simulink model "track_vehicle_EKF1"  (R2017b)
settings: Solver=ode45  StartTime=0.0  StopTime=300  FixedStep=0.1  RelTol=1e-3  EnableMultiTasking=on
PreLoadFcn:
  | RTWConfigurationCB('preloadfcn', bdroot);
InitFcn:
  | parameterVehicle
  | parameterGNC
StopFcn:
  | myAnimation(xActEst,yActEst,thetaActEst,X_array,Y_array,rp1,rp2)
  | myStopFcn2sim(xActEst,yActEst,X_array,Y_array,rp1,rp2)
undefined symbols (not defined in the file): bDR, dcArrayC, DiscIntNeverNeededParam, Earth, eTickDR, KP1, KP2, rNominalDR, rp1, rp2, Tau1, Tau2, TauEncoderDR, Tsample, TsampleEncoderDR, Vcom, wArrayC, WGS84, X, X_array, Y, Y_array
libraries: simulink x12, robotlib x8, aerolibtransform2 x1, dspsigops x1, aerolibanimutils x1
CloseFcn:
  | rtwprivate ssgencode ModelCloseRequest track_vehicle6_v2
settings Model: Creator=Dogan  LastModifiedBy=ayushi
settings DataIOCC: LimitDataPoints=on  SaveFormat=Array  SignalLoggingSaveFormat=ModelDataLogs
settings OptimizationCC: ExpressionDepthLimit=2147483647  InitFltsAndDblsToZero=on  LifeSpan=inf
settings DebuggingCC: SaveWithParameterizedLinksMsg=none  UnderspecifiedInitializationDetection=Classic  MergeDetectMultiDrivingBlocksExec=none  SignalResolutionControl=TryResolveAllWithWarning  SolverPrmCheckMsg=warning  MultiTaskDSMMsg=warning  MultiTaskCondExecSysMsg=none  ParameterPrecisionLossMsg=none  FcnCallInpInsideContextMsg=warning  StateNameClashWarn=warning  SFUnexpectedBacktrackingDiag=warning  SFNoUnconditionalDefaultTransitionDiag=warning  SFExecutionAtInitializationDiag=none
settings HardwareCC: ProdBitPerLong=64  ProdLargestAtomicFloat=None  ProdHWDeviceType=Intel->x86-64  TargetHWDeviceType=32-bit Generic
settings ModelReferenceCC: PropagateSignalLabelsOutOfModel=off
settings SFSimCC: SimParseCustomCode=off
settings RTWCC: Description=Generic Real-Time Target
settings CodeAppCC: GenerateComments=off  SimulinkBlockComments=off
settings GRTTargetCC: TargetLangStandard=C89/C90 (ANSI)  GeneratePreprocessorConditionals=Disable all
settings ConfigComp: CovMetricSettings=dw  CovHtmlReporting=on  CovSaveCumulativeToWorkspaceVar=on  CovSaveSingleToWorkspaceVar=on  CovExternalEMLEnable=off

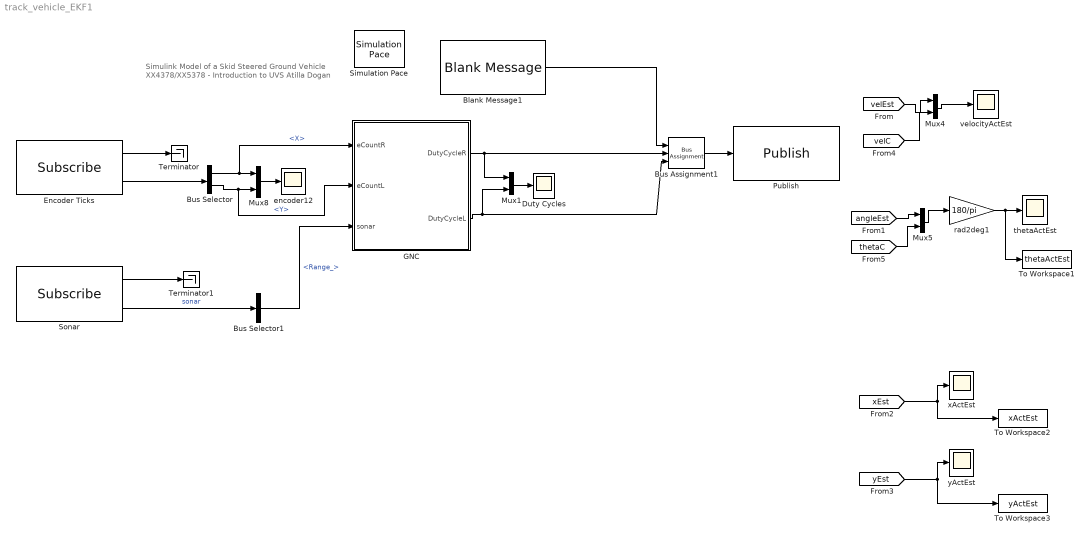
== system track_vehicle_EKF1 ==
  note: Simulink Model of a Skid Steered Ground Vehicle
      | XX4378/XX5378 - Introduction to UVS
      | Atilla Dogan
  Blank Message1 : robotlib/Blank Message  SourceLibraryInfo=This block requires Robotics System Toolbox  messageType=geometry_msgs/Point  SampleTime=inf
      settings: SourceProductBaseCode=RO
  Bus Assignment1 : BusAssignment  AssignedSignals=X,Y
  Bus Selector : BusSelector  OutputSignals=Point.X,Point.Y
  Bus Selector1 : BusSelector  OutputSignals=Range_
  Duty Cycles : Scope
  Encoder Ticks : robotlib/Subscribe  SourceLibraryInfo=This block requires Robotics System Toolbox  topicSource=Select from ROS network  topic=/enc  messageType=geometry_msgs/PointStamped  sampleTime=-1  messageQueueLength=1
      settings: SourceProductBaseCode=RO
  GNC : Subsystem
  Mux{1,4..5,8} (4 alike) : Mux  Inputs=2
  Publish : robotlib/Publish  SourceLibraryInfo=This block requires Robotics System Toolbox  topicSource=Select from ROS network  topic=/cmd_pwm  messageType=geometry_msgs/Point  messageQueueLength=10
      settings: SourceProductBaseCode=RO
  Simulation Pace : aerolibanimutils/Simulation Pace  SimulationPace=1  SleepMode=MATLAB Thread  OutputPaceError=off  SampleTime=1/30
  Sonar : robotlib/Subscribe  SourceLibraryInfo=This block requires Robotics System Toolbox  topicSource=Select from ROS network  topic=/mavros/distance_sensor/hrlv_ez4_pub  messageType=sensor_msgs/Range  sampleTime=-1  messageQueueLength=1
      settings: SourceProductBaseCode=RO
  Terminator : Terminator
  Terminator1 : Terminator
  To Workspace1 : ToWorkspace  VariableName=thetaActEst  SaveFormat=Structure With Time  SampleTime=-1
  To Workspace2 : ToWorkspace  VariableName=xActEst  SaveFormat=Structure With Time  SampleTime=-1
  To Workspace3 : ToWorkspace  VariableName=yActEst  SaveFormat=Structure With Time  SampleTime=-1
  encoder12 : Scope
  rad2deg1 : Gain  Gain=180/pi
  thetaActEst : Scope
  velocityActEst : Scope
  xActEst : Scope
  yActEst : Scope
  wires:
  GNC/1(DutyCycleR) -> Bus Assignment1/2, Mux1/1
  GNC/2(DutyCycleL) -> Bus Assignment1/3, Mux1/2
  Mux1/1 -> Duty Cycles/1
  Mux4/1 -> velocityActEst/1
  [velEst] -> Mux4/1
  rad2deg1/1 -> To Workspace1/1, thetaActEst/1
  Mux5/1 -> rad2deg1/1
  [angleEst] -> Mux5/1
  [xEst] -> xActEst/1, To Workspace2/1
  [yEst] -> yActEst/1, To Workspace3/1
  [velC] -> Mux4/2
  [thetaC] -> Mux5/2
  Encoder Ticks/2 -> Bus Selector/1
  Bus Selector/2 -> GNC/2(eCountL), Mux8/2  "<Y>"
  Bus Selector/1 -> GNC/1(eCountR), Mux8/1  "<X>"
  Mux8/1 -> encoder12/1
  Encoder Ticks/1 -> Terminator/1
  Blank Message1/1 -> Bus Assignment1/1
  Bus Assignment1/1 -> Publish/1
  Sonar/1 -> Terminator1/1
  Sonar/2 -> Bus Selector1/1  "sonar"
  Bus Selector1/1 -> GNC/3(sonar)  "<Range_>"

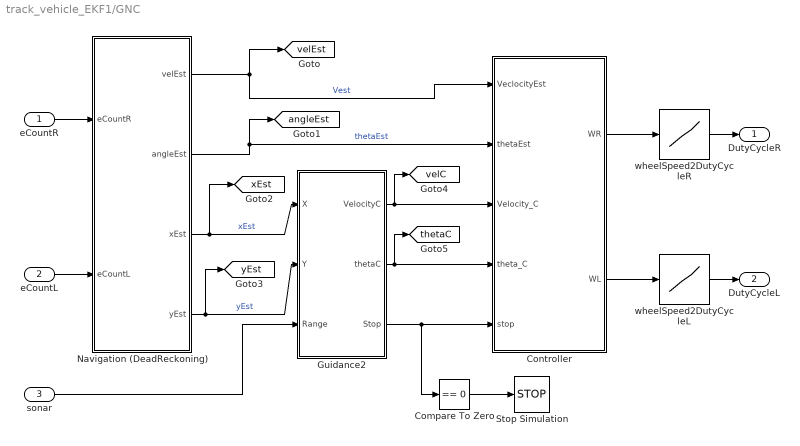
== system track_vehicle_EKF1/GNC ==
  eCountR : Inport
  eCountL : Inport  Port=2
  sonar : Inport  Port=3
  Compare To Zero : simulink/Logic and Bit Operations/Compare To Zero  relop===  OutDataTypeStr=boolean
  Controller : Subsystem
  Guidance2 : Subsystem
  Navigation (DeadReckoning) : Subsystem
  Stop Simulation : Stop
  wheelSpeed2DutyCycleL : Lookup  InputValues=wArrayC  Table=dcArrayC  LookUpMeth=Use Input Nearest
  wheelSpeed2DutyCycleR : Lookup  InputValues=wArrayC  Table=dcArrayC  LookUpMeth=Use Input Nearest
  DutyCycleR : Outport
  DutyCycleL : Outport  Port=2
  tag scope: angleEst=global, thetaC=global, velC=global, velEst=global, xEst=global, yEst=global
  wires:
  Guidance2/3(Stop) -> Compare To Zero/1, Controller/5(stop)
  Controller/1(WR) -> wheelSpeed2DutyCycleR/1
  Navigation (DeadReckoning)/4(yEst) -> [yEst], Guidance2/2(Y)  "yEst"
  Navigation (DeadReckoning)/3(xEst) -> Guidance2/1(X), [xEst]  "xEst"
  Navigation (DeadReckoning)/2(angleEst) -> Controller/2(thetaEst), [angleEst]  "thetaEst"
  Navigation (DeadReckoning)/1(velEst) -> Controller/1(VeclocityEst), [velEst]  "Vest"
  eCountL/1 -> Navigation (DeadReckoning)/2(eCountL)
  eCountR/1 -> Navigation (DeadReckoning)/1(eCountR)
  Guidance2/1(VelocityC) -> Controller/3(Velocity_C), [velC]
  Guidance2/2(thetaC) -> Controller/4(theta_C), [thetaC]
  wheelSpeed2DutyCycleR/1 -> DutyCycleR/1
  Controller/2(WL) -> wheelSpeed2DutyCycleL/1
  wheelSpeed2DutyCycleL/1 -> DutyCycleL/1
  Compare To Zero/1 -> Stop Simulation/1
  sonar/1 -> Guidance2/3(Range)

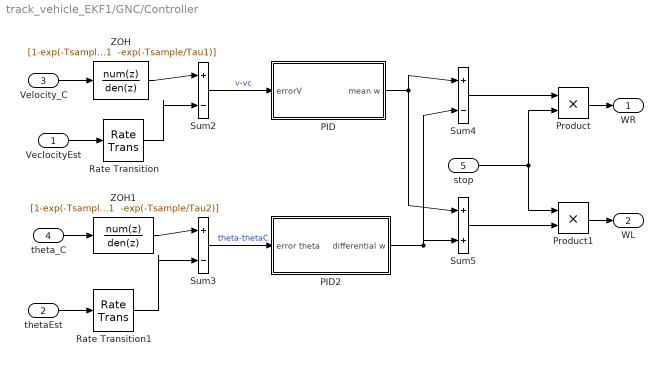
== system track_vehicle_EKF1/GNC/Controller ==
  VeclocityEst : Inport
  thetaEst : Inport  Port=2
  Velocity_C : Inport  Port=3
  theta_C : Inport  Port=4
  stop : Inport  Port=5
  PID : Subsystem
  PID2 : Subsystem
  Product : Product  RndMeth=Zero
  Product1 : Product  RndMeth=Zero
  Rate Transition : RateTransition  Deterministic=off
  Rate Transition1 : RateTransition  Deterministic=off
  Sum2 : Sum  Inputs=|+|-|  SampleTime=Tsample
  Sum3 : Sum  Inputs=|+|-|  SampleTime=Tsample
  Sum4 : Sum  Inputs=+|-
  Sum5 : Sum  Inputs=+|+
  ZOH : DiscreteTransferFcn  Numerator=[1-exp(-Tsample/Tau1)]  Denominator="[1  -exp(-Tsample/Tau1)]"  SampleTime=Tsample
  ZOH1 : DiscreteTransferFcn  Numerator=[1-exp(-Tsample/Tau2)]  Denominator="[1  -exp(-Tsample/Tau2)]"  SampleTime=Tsample
  WR : Outport
  WL : Outport  Port=2
  wires:
  Product1/1 -> WL/1
  Product/1 -> WR/1
  Sum5/1 -> Product1/2
  stop/1 -> Product/2, Product1/1
  Sum4/1 -> Product/1
  PID2/1(differential w) -> Sum5/2, Sum4/2
  PID/1(mean w) -> Sum5/1, Sum4/1
  theta_C/1 -> ZOH1/1
  thetaEst/1 -> Rate Transition1/1
  Velocity_C/1 -> ZOH/1
  VeclocityEst/1 -> Rate Transition/1
  Sum2/1 -> PID/1(errorV)  "v-vc"
  Sum3/1 -> PID2/1(error theta)  "theta-thetaC"
  ZOH/1 -> Sum2/1
  Rate Transition/1 -> Sum2/2
  ZOH1/1 -> Sum3/1
  Rate Transition1/1 -> Sum3/2

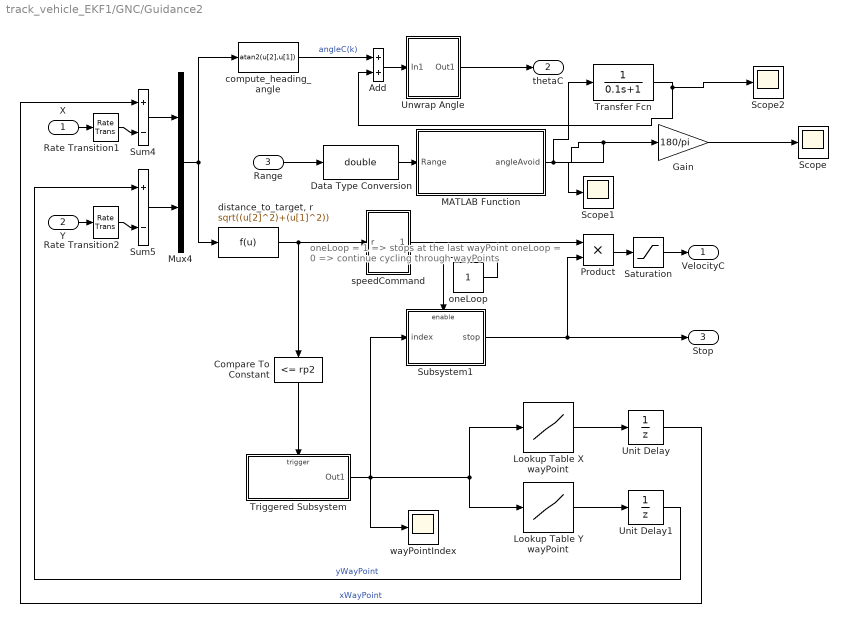
== system track_vehicle_EKF1/GNC/Guidance2 ==
  note: oneLoop = 1 => stops at the last wayPoint
      | oneLoop = 0 => continue cycling through wayPoints
  X : Inport
  Y : Inport  Port=2
  Range : Inport  Port=3
  Add : Sum
  Compare To Constant : simulink/Logic and Bit Operations/Compare To Constant  relop=<=  const=rp2  OutDataTypeStr=uint8  ZeroCross=off
  Data Type Conversion : DataTypeConversion  OutDataTypeStr=double
  Gain : Gain  Gain=180/pi
  Lookup Table X wayPoint : Lookup  InputValues=[1:length(X_array)]  Table=X_array  LookUpMeth=Interpolation-Use End Values  OutDataTypeStr=double
  Lookup Table Y wayPoint : Lookup  InputValues=[1:length(Y_array)]  Table=Y_array  LookUpMeth=Interpolation-Use End Values  OutDataTypeStr=double
  MATLAB Function : MATLAB Function  TreatAsAtomicUnit=on
  Mux4 : Mux  Inputs=2
  Product : Product  RndMeth=Zero
  Rate Transition1 : RateTransition
  Rate Transition2 : RateTransition
  Saturation : Saturate  UpperLimit=Vcom  LowerLimit=0  SampleTime=Tsample
  Scope : Scope
  Scope1 : Scope
  Scope2 : Scope
  Subsystem1 : Subsystem
  Sum4 : Sum  Inputs=|+|-|
  Sum5 : Sum  Inputs=|+|-|
  Transfer Fcn : TransferFcn  Denominator=[0.1 1]
  Triggered Subsystem : Subsystem  TreatAsAtomicUnit=on
  Unit Delay : UnitDelay  SampleTime=Tsample
  Unit Delay1 : UnitDelay  SampleTime=Tsample
  Unwrap Angle : Subsystem
  compute_heading_angle : Fcn  Expr=atan2(u[2],u[1])  SampleTime=Tsample
  "distance_to_target, r" : Fcn  Expr=sqrt((u[2]^2)+(u[1]^2))  SampleTime=Tsample
  oneLoop : Constant  OutDataTypeStr=uint32  SampleTime=Tsample
  speedCommand : Subsystem
  wayPointIndex : Scope
  VelocityC : Outport
  thetaC : Outport  Port=2
  Stop : Outport  Port=3
  wires:
  speedCommand/1(Vdes) -> Product/1
  compute_heading_angle/1 -> Add/1  "angleC(k)"
  Sum4/1 -> Mux4/1
  "distance_to_target, r"/1 -> speedCommand/1(r), Compare To Constant/1
  Mux4/1 -> "distance_to_target, r"/1, compute_heading_angle/1
  Lookup Table X wayPoint/1 -> Unit Delay/1
  Lookup Table Y wayPoint/1 -> Unit Delay1/1
  X/1 -> Rate Transition1/1
  Y/1 -> Rate Transition2/1
  Sum5/1 -> Mux4/2
  Compare To Constant/1 -> Triggered Subsystem/Trigger
  Triggered Subsystem/1(Out1) -> Subsystem1/1(index), wayPointIndex/1, Lookup Table X wayPoint/1, Lookup Table Y wayPoint/1
  Unit Delay/1 -> Sum4/1  "xWayPoint"
  Unit Delay1/1 -> Sum5/1  "yWayPoint"
  Saturation/1 -> VelocityC/1
  Unwrap Angle/1(Out1) -> thetaC/1
  Rate Transition1/1 -> Sum4/2
  Rate Transition2/1 -> Sum5/2
  Product/1 -> Saturation/1
  Subsystem1/1(stop) -> Product/2, Stop/1
  oneLoop/1 -> Subsystem1/Enable
  Gain/1 -> Scope/1
  Data Type Conversion/1 -> MATLAB Function/1(Range)
  Range/1 -> Data Type Conversion/1
  Add/1 -> Unwrap Angle/1(In1)
  MATLAB Function/1(angleAvoid) -> Transfer Fcn/1, Scope1/1, Gain/1
  Transfer Fcn/1 -> Scope2/1, Add/2

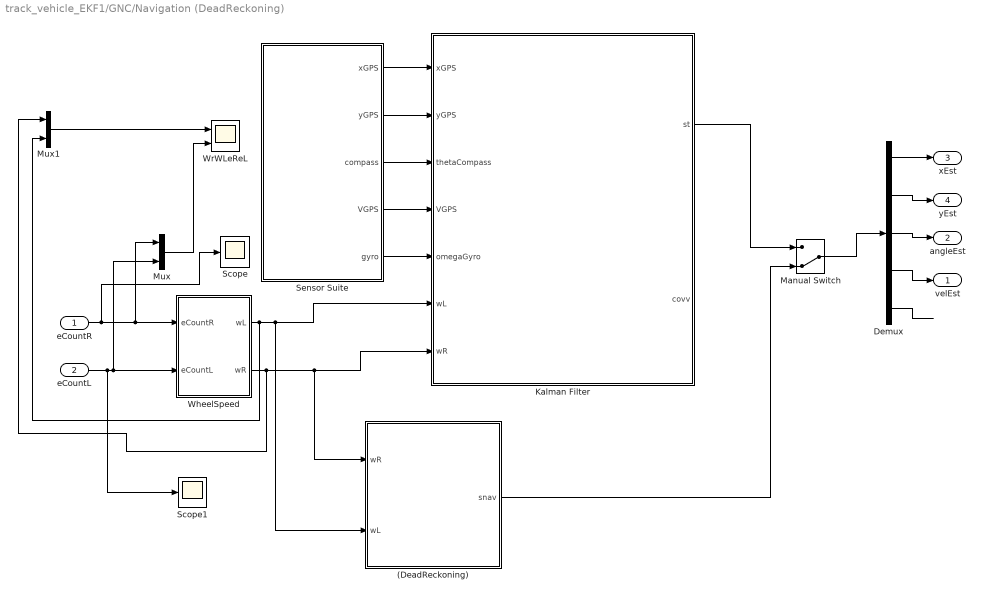
== system track_vehicle_EKF1/GNC/Navigation (DeadReckoning) ==
  eCountR : Inport
  eCountL : Inport  Port=2
  (DeadReckoning) : Subsystem
  Demux : Demux  Outputs=5
  Kalman Filter : MATLAB Function  TreatAsAtomicUnit=on  SystemSampleTime=Tsample
  Manual Switch : ManualSwitch  CurrentSetting=0
  Mux : Mux  Inputs=2
  Mux1 : Mux  Inputs=2
  Scope : Scope
  Scope1 : Scope
  Sensor Suite : Subsystem
  WheelSpeed : Subsystem
  WrWLeReL : Scope  NumInputPorts=2
  velEst : Outport
  angleEst : Outport  Port=2
  xEst : Outport  Port=3
  yEst : Outport  Port=4
  wires:
  WheelSpeed/2(wR) -> Mux1/1, (DeadReckoning)/1(wR), Kalman Filter/7(wR)
  eCountL/1 -> Scope1/1, WheelSpeed/2(eCountL), Mux/2
  eCountR/1 -> Scope/1, Mux/1, WheelSpeed/1(eCountR)
  Sensor Suite/5(gyro) -> Kalman Filter/5(omegaGyro)
  Demux/5 -> ?
  Demux/1 -> xEst/1
  Demux/2 -> yEst/1
  Demux/3 -> angleEst/1
  Demux/4 -> velEst/1
  Kalman Filter/1(st) -> Manual Switch/1
  (DeadReckoning)/1(snav) -> Manual Switch/2
  Manual Switch/1 -> Demux/1
  WheelSpeed/1(wL) -> Kalman Filter/6(wL), (DeadReckoning)/2(wL), Mux1/2
  Mux/1 -> WrWLeReL/2
  Mux1/1 -> WrWLeReL/1
  Sensor Suite/1(xGPS) -> Kalman Filter/1(xGPS)
  Sensor Suite/2(yGPS) -> Kalman Filter/2(yGPS)
  Sensor Suite/3(compass) -> Kalman Filter/3(thetaCompass)
  Sensor Suite/4(VGPS) -> Kalman Filter/4(VGPS)

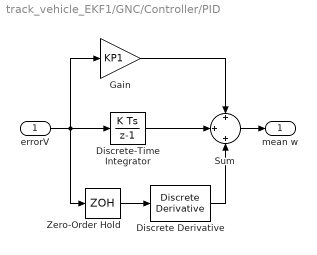
== system track_vehicle_EKF1/GNC/Controller/PID ==
  errorV : Inport
  Discrete Derivative : simulink/Discrete/Discrete Derivative  gainval=KD1  ICPrevScaledInput=0.0  InputProcessing=Inherited  OutMin=[]  OutMax=[]  OutDataType=sfix(16)  OutScaling=2^-10  DoSatur=off
  Discrete-Time Integrator : DiscreteIntegrator  gainval=KI1  SampleTime=Tsample  ICPrevOutput=DiscIntNeverNeededParam  ICPrevScaledInput=DiscIntNeverNeededParam
  Gain : Gain  Gain=KP1  SampleTime=Tsample
  Sum : Sum  Inputs=+|+|+
  Zero-Order Hold : ZeroOrderHold  SampleTime=Tsample
  mean w : Outport
  wires:
  Discrete Derivative/1 -> Sum/3
  Zero-Order Hold/1 -> Discrete Derivative/1
  Discrete-Time Integrator/1 -> Sum/2
  Gain/1 -> Sum/1
  errorV/1 -> Discrete-Time Integrator/1, Gain/1, Zero-Order Hold/1
  Sum/1 -> mean w/1

== system track_vehicle_EKF1/GNC/Controller/PID2 ==
  error theta : Inport
  Discrete Derivative1 : simulink/Discrete/Discrete Derivative  gainval=KD2  ICPrevScaledInput=0.0  InputProcessing=Inherited  OutMin=[]  OutMax=[]  OutDataType=sfix(16)  OutScaling=2^-10  DoSatur=off
  Discrete-Time Integrator1 : DiscreteIntegrator  gainval=KI2  SampleTime=Tsample  ICPrevOutput=DiscIntNeverNeededParam  ICPrevScaledInput=DiscIntNeverNeededParam
  Gain1 : Gain  Gain=KP2  SampleTime=Tsample
  Sum1 : Sum  Inputs=+|+|+
  Zero-Order Hold1 : ZeroOrderHold  SampleTime=Tsample
  differential w : Outport
  wires:
  Discrete Derivative1/1 -> Sum1/3
  Zero-Order Hold1/1 -> Discrete Derivative1/1
  error theta/1 -> Gain1/1, Discrete-Time Integrator1/1, Zero-Order Hold1/1
  Discrete-Time Integrator1/1 -> Sum1/2
  Gain1/1 -> Sum1/1
  Sum1/1 -> differential w/1

== system track_vehicle_EKF1/GNC/Guidance2/Subsystem1 ==
  note: NAND = TRUE
      | if at least one input is FALSE
  index : Inport
  Enable : EnablePort
  Compare To Constant1 : simulink/Logic and Bit Operations/Compare To Constant  relop===  const=1  OutDataTypeStr=uint8  ZeroCross=off
  Compare To Constant2 : simulink/Logic and Bit Operations/Compare To Constant  relop===  const=length(X_array)  OutDataTypeStr=uint8  ZeroCross=off
  Logical Operator1 : Logic  Operator=NAND  IconShape=distinctive  AllPortsSameDT=off  OutDataTypeStr=boolean
  Triggered Subsystem2 : Subsystem  TreatAsAtomicUnit=on
  stop : Outport  OutputWhenDisabled=reset  InitialOutput=[1]
  wires:
  Logical Operator1/1 -> stop/1
  index/1 -> Compare To Constant1/1, Compare To Constant2/1
  Compare To Constant1/1 -> Logical Operator1/1
  Triggered Subsystem2/1(Out1) -> Logical Operator1/2
  Compare To Constant2/1 -> Triggered Subsystem2/Trigger

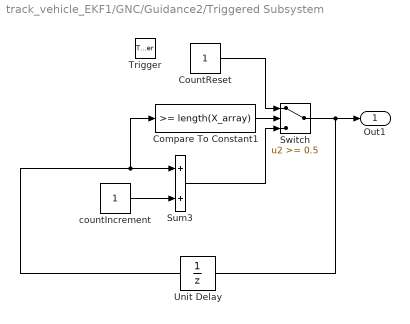
== system track_vehicle_EKF1/GNC/Guidance2/Triggered Subsystem ==
  Trigger : TriggerPort  VariantControl=(inherit)
  Compare To Constant1 : simulink/Logic and Bit Operations/Compare To Constant  relop=>=  const=length(X_array)  OutDataTypeStr=uint8  ZeroCross=off
  CountReset : Constant  OutDataTypeStr=uint32  SampleTime=-1
  Sum3 : Sum  OutDataTypeStr=uint32
  Switch : Switch  Threshold=0.5
  Unit Delay : UnitDelay  InitialCondition=1  SampleTime=-1
  countIncrement : Constant  OutDataTypeStr=uint32  SampleTime=-1
  Out1 : Outport  OutDataTypeStr=uint32  InitialOutput=1
  wires:
  countIncrement/1 -> Sum3/2
  Unit Delay/1 -> Sum3/1, Compare To Constant1/1
  Compare To Constant1/1 -> Switch/2
  Switch/1 -> Out1/1, Unit Delay/1
  CountReset/1 -> Switch/1
  Sum3/1 -> Switch/3

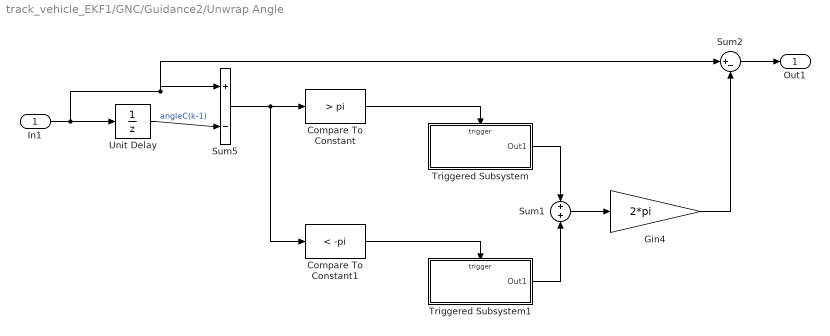
== system track_vehicle_EKF1/GNC/Guidance2/Unwrap Angle ==
  In1 : Inport
  Compare To Constant : simulink/Logic and Bit Operations/Compare To Constant  relop=>  const=pi  OutDataTypeStr=uint8  ZeroCross=off
  Compare To Constant1 : simulink/Logic and Bit Operations/Compare To Constant  relop=<  const=-pi  OutDataTypeStr=uint8  ZeroCross=off
  Gin4 : Gain  Gain=2*pi  OutDataTypeStr=double  SampleTime=Tsample
  Sum1 : Sum  Inputs=+|+
  Sum2 : Sum  Inputs=|+-
  Sum5 : Sum  Inputs=|+|-|
  Triggered Subsystem : Subsystem  TreatAsAtomicUnit=on
  Triggered Subsystem1 : Subsystem  TreatAsAtomicUnit=on
  Unit Delay : UnitDelay  SampleTime=Tsample
  Out1 : Outport
  wires:
  In1/1 -> Unit Delay/1, Sum5/1, Sum2/1
  Unit Delay/1 -> Sum5/2  "angleC(k-1)"
  Sum5/1 -> Compare To Constant/1, Compare To Constant1/1
  Compare To Constant1/1 -> Triggered Subsystem1/Trigger
  Compare To Constant/1 -> Triggered Subsystem/Trigger
  Triggered Subsystem/1(Out1) -> Sum1/1
  Triggered Subsystem1/1(Out1) -> Sum1/2
  Sum1/1 -> Gin4/1
  Sum2/1 -> Out1/1
  Gin4/1 -> Sum2/2

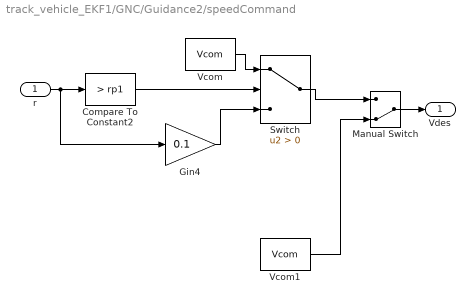
== system track_vehicle_EKF1/GNC/Guidance2/speedCommand ==
  r : Inport
  Compare To Constant2 : simulink/Logic and Bit Operations/Compare To Constant  relop=>  const=rp1  OutDataTypeStr=uint8  ZeroCross=off
  Gin4 : Gain  Gain=0.1  SampleTime=Tsample
  Manual Switch : ManualSwitch  CurrentSetting=0
  Switch : Switch  Criteria=u2 > Threshold
  Vcom : Constant  Value=Vcom  SampleTime=Tsample
  Vcom1 : Constant  Value=Vcom  SampleTime=Tsample
  Vdes : Outport
  wires:
  Compare To Constant2/1 -> Switch/2
  Vcom/1 -> Switch/1
  Vcom1/1 -> Manual Switch/2
  Switch/1 -> Manual Switch/1
  Gin4/1 -> Switch/3
  r/1 -> Compare To Constant2/1, Gin4/1
  Manual Switch/1 -> Vdes/1

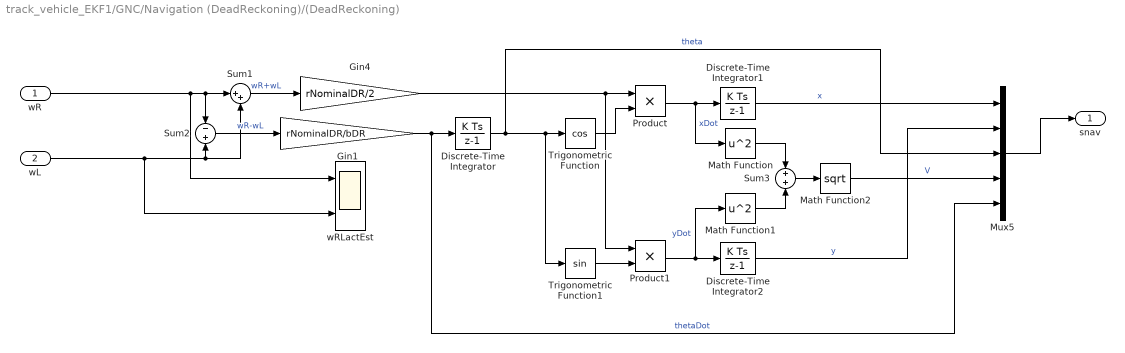
== system track_vehicle_EKF1/GNC/Navigation (DeadReckoning)/(DeadReckoning) ==
  wR : Inport
  wL : Inport  Port=2
  Discrete-Time Integrator : DiscreteIntegrator  SampleTime=TsampleEncoderDR  ICPrevOutput=DiscIntNeverNeededParam  ICPrevScaledInput=DiscIntNeverNeededParam
  Discrete-Time Integrator1 : DiscreteIntegrator  SampleTime=TsampleEncoderDR  ICPrevOutput=DiscIntNeverNeededParam  ICPrevScaledInput=DiscIntNeverNeededParam
  Discrete-Time Integrator2 : DiscreteIntegrator  SampleTime=TsampleEncoderDR  ICPrevOutput=DiscIntNeverNeededParam  ICPrevScaledInput=DiscIntNeverNeededParam
  Gin1 : Gain  Gain=rNominalDR/bDR  OutDataTypeStr=double
  Gin4 : Gain  Gain=rNominalDR/2  OutDataTypeStr=double
  Math Function : Math  Operator=square  SaturateOnIntegerOverflow=on
  Math Function1 : Math  Operator=square  SaturateOnIntegerOverflow=on
  Math Function2 : Math  Operator=sqrt  OutputSignalType=real  SaturateOnIntegerOverflow=on
  Mux5 : Mux  Inputs=5
  Product : Product  RndMeth=Zero
  Product1 : Product  RndMeth=Zero
  Sum1 : Sum  Inputs=|++
  Sum2 : Sum  Inputs=-|+
  Sum3 : Sum  Inputs=+|+
  Trigonometric Function : Trigonometry  Operator=cos  OutputSignalType=real
  Trigonometric Function1 : Trigonometry  OutputSignalType=real
  wRLactEst : Scope  NumInputPorts=2
  snav : Outport
  wires:
  wL/1 -> Sum2/2, Sum1/2, wRLactEst/2
  wR/1 -> Sum2/1, Sum1/1, wRLactEst/1
  Math Function2/1 -> Mux5/4  "V"
  Sum3/1 -> Math Function2/1
  Math Function1/1 -> Sum3/2
  Math Function/1 -> Sum3/1
  Discrete-Time Integrator2/1 -> Mux5/2  "y"
  Discrete-Time Integrator1/1 -> Mux5/1  "x"
  Product1/1 -> Math Function1/1, Discrete-Time Integrator2/1  "yDot"
  Product/1 -> Math Function/1, Discrete-Time Integrator1/1  "xDot"
  Trigonometric Function1/1 -> Product1/2
  Gin4/1 -> Product1/1, Product/1
  Trigonometric Function/1 -> Product/2
  Discrete-Time Integrator/1 -> Mux5/3, Trigonometric Function1/1, Trigonometric Function/1  "theta"
  Gin1/1 -> Mux5/5, Discrete-Time Integrator/1  "thetaDot"
  Sum2/1 -> Gin1/1  "wR-wL"
  Sum1/1 -> Gin4/1  "wR+wL"
  Mux5/1 -> snav/1

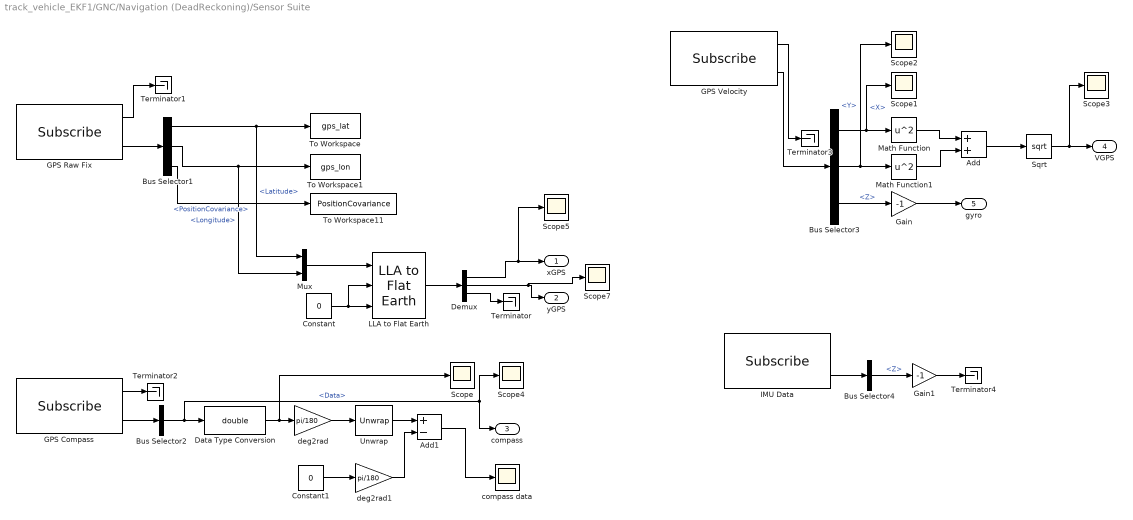
== system track_vehicle_EKF1/GNC/Navigation (DeadReckoning)/Sensor Suite ==
  " GPS Compass" : robotlib/Subscribe  SourceLibraryInfo=This block requires Robotics System Toolbox  topicSource=Select from ROS network  topic=/mavros/global_position/compass_hdg  messageType=std_msgs/Float64  sampleTime=-1  messageQueueLength=1
      settings: SourceProductBaseCode=RO
  Add : Sum  Inputs=2
  Add1 : Sum  Inputs=+-
  Bus Selector1 : BusSelector  OutputSignals=Latitude,Longitude,PositionCovariance
  Bus Selector2 : BusSelector  OutputSignals=Data
  Bus Selector3 : BusSelector  OutputSignals=Twist.Linear.X,Twist.Linear.Y,Twist.Angular.Z
  Bus Selector4 : BusSelector  OutputSignals=AngularVelocity.Z
  Constant : Constant  Value=0
  Constant1 : Constant  Value=0
  Data Type Conversion : DataTypeConversion  OutDataTypeStr=double
  Demux : Demux  Outputs=3
  GPS Raw Fix : robotlib/Subscribe  SourceLibraryInfo=This block requires Robotics System Toolbox  topicSource=Select from ROS network  topic=/mavros/global_position/raw/fix  messageType=sensor_msgs/NavSatFix  sampleTime=-1  messageQueueLength=1
      settings: SourceProductBaseCode=RO
  "GPS Velocity " : robotlib/Subscribe  SourceLibraryInfo=This block requires Robotics System Toolbox  topicSource=Select from ROS network  topic=/mavros/global_position/raw/gps_vel  messageType=geometry_msgs/TwistStamped  sampleTime=-1  messageQueueLength=1
      settings: SourceProductBaseCode=RO
  Gain : Gain  Gain=-1
  Gain1 : Gain  Gain=-1
  IMU Data : robotlib/Subscribe  SourceLibraryInfo=This block requires Robotics System Toolbox  topicSource=Select from ROS network  topic=/mavros/imu/data  messageType=sensor_msgs/Imu  sampleTime=-1  messageQueueLength=1
      settings: SourceProductBaseCode=RO
  LLA to Flat Earth : aerolibtransform2/LLA to Flat Earth  units=Metric (MKS)  ptype=Earth (WGS84)  F=1/298.257223563  R=6378137  LL0=[32.7336 -97.1169]  psi=0
      settings: SourceProductName=Aerospace Blockset  SourceProductBaseCode=AE
  Math Function : Math  Operator=square  SaturateOnIntegerOverflow=on
  Math Function1 : Math  Operator=square  SaturateOnIntegerOverflow=on
  Mux : Mux  Inputs=2
  Scope{,1..5,7} (7 alike) : Scope
  Sqrt : Sqrt  SaturateOnIntegerOverflow=on
  Terminator{,1..4} (5 alike) : Terminator
  To Workspace : ToWorkspace  VariableName=gps_lat  SaveFormat=Timeseries  SampleTime=-1
  To Workspace1 : ToWorkspace  VariableName=gps_lon  SaveFormat=Timeseries  SampleTime=-1
  To Workspace11 : ToWorkspace  VariableName=PositionCovariance  SaveFormat=Timeseries  SampleTime=-1
  Unwrap : dspsigops/Unwrap  tol=pi  InputProcessing=Columns as channels (frame based)  running=off
  compass data : Scope
  deg2rad : Gain  Gain=pi/180
  deg2rad1 : Gain  Gain=pi/180
  xGPS : Outport
  yGPS : Outport  Port=2
  compass : Outport  Port=3
  VGPS : Outport  Port=4
  gyro : Outport  Port=5
  wires:
  GPS Raw Fix/2 -> Bus Selector1/1
  Bus Selector1/1 -> To Workspace/1, Mux/1  "<Latitude>"
  " GPS Compass"/2 -> Bus Selector2/1
  Bus Selector1/2 -> Mux/2, To Workspace1/1  "<Longitude>"
  Mux/1 -> LLA to Flat Earth/1
  Constant/1 -> LLA to Flat Earth/3, LLA to Flat Earth/2
  LLA to Flat Earth/1 -> Demux/1
  Demux/1 -> Scope5/1, xGPS/1
  Demux/2 -> Scope7/1, yGPS/1
  Bus Selector1/3 -> To Workspace11/1  "<PositionCovariance>"
  "GPS Velocity "/2 -> Bus Selector3/1
  Bus Selector3/1 -> Scope1/1, Math Function/1  "<X>"
  Bus Selector3/2 -> Scope2/1, Math Function1/1  "<Y>"
  Math Function1/1 -> Add/2
  Math Function/1 -> Add/1
  Add/1 -> Sqrt/1
  Sqrt/1 -> Scope3/1, VGPS/1
  Bus Selector3/3 -> Gain/1  "<Z>"
  Demux/3 -> Terminator/1
  GPS Raw Fix/1 -> Terminator1/1
  " GPS Compass"/1 -> Terminator2/1
  "GPS Velocity "/1 -> Terminator3/1
  IMU Data/2 -> Bus Selector4/1
  Bus Selector2/1 -> compass/1, Scope4/1, Data Type Conversion/1  "<Data>"
  Data Type Conversion/1 -> Scope/1, deg2rad/1
  deg2rad/1 -> Unwrap/1
  Constant1/1 -> deg2rad1/1
  Unwrap/1 -> Add1/1
  deg2rad1/1 -> Add1/2
  Add1/1 -> compass data/1
  Bus Selector4/1 -> Gain1/1  "<Z>"
  Gain1/1 -> Terminator4/1
  Gain/1 -> gyro/1

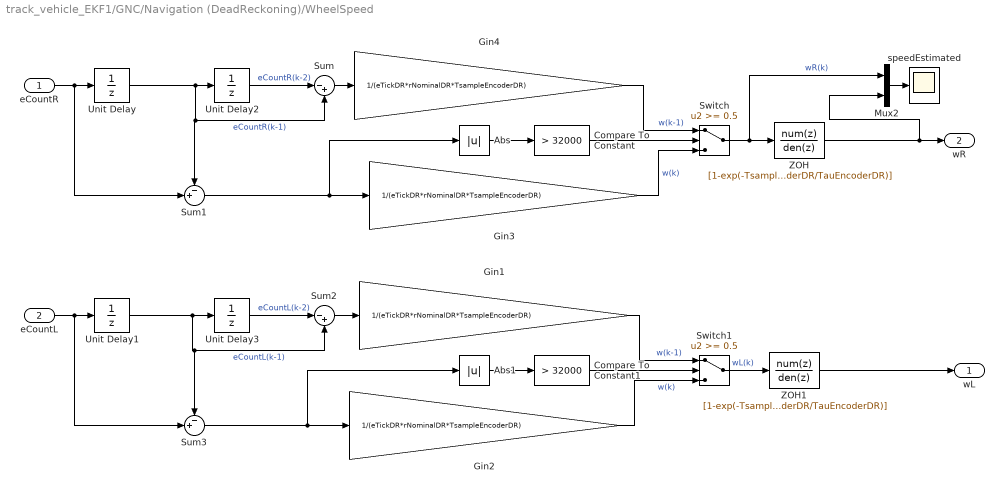
== system track_vehicle_EKF1/GNC/Navigation (DeadReckoning)/WheelSpeed ==
  eCountR : Inport
  eCountL : Inport  Port=2
  Abs : Abs
  Abs1 : Abs
  Compare To Constant : simulink/Logic and Bit Operations/Compare To Constant  relop=>  const=32000  OutDataTypeStr=uint8  ZeroCross=off
  Compare To Constant1 : simulink/Logic and Bit Operations/Compare To Constant  relop=>  const=32000  OutDataTypeStr=uint8  ZeroCross=off
  Gin{1..4} (4 alike) : Gain  Gain=1/(eTickDR*rNominalDR*TsampleEncoderDR)  OutDataTypeStr=double  SampleTime=TsampleEncoderDR
  Mux2 : Mux  Inputs=2
  Sum : Sum  Inputs=|-+
  Sum1 : Sum  Inputs=-+|
  Sum2 : Sum  Inputs=|-+
  Sum3 : Sum  Inputs=-+|
  Switch : Switch  Threshold=0.5
  Switch1 : Switch  Threshold=0.5
  Unit Delay{,1..3} (4 alike) : UnitDelay  SampleTime=TsampleEncoderDR
  ZOH : DiscreteTransferFcn  Numerator=[1-exp(-TsampleEncoderDR/TauEncoderDR)]  Denominator="[1  -exp(-TsampleEncoderDR/TauEncoderDR)]"  SampleTime=TsampleEncoderDR
  ZOH1 : DiscreteTransferFcn  Numerator=[1-exp(-TsampleEncoderDR/TauEncoderDR)]  Denominator="[1  -exp(-TsampleEncoderDR/TauEncoderDR)]"  SampleTime=TsampleEncoderDR
  speedEstimated : Scope
  wL : Outport
  wR : Outport  Port=2
  wires:
  Mux2/1 -> speedEstimated/1
  ZOH1/1 -> wL/1
  ZOH/1 -> wR/1, Mux2/2
  Switch1/1 -> ZOH1/1  "wL(k)"
  Switch/1 -> Mux2/1, ZOH/1  "wR(k)"
  Compare To Constant1/1 -> Switch1/2
  Abs1/1 -> Compare To Constant1/1
  Gin2/1 -> Switch1/3  "w(k)"
  Gin1/1 -> Switch1/1  "w(k-1)"
  Sum3/1 -> Gin2/1, Abs1/1
  Sum2/1 -> Gin1/1
  Unit Delay3/1 -> Sum2/1  "eCountL(k-2)"
  Unit Delay1/1 -> Unit Delay3/1, Sum2/2, Sum3/1  "eCountL(k-1)"
  eCountL/1 -> Unit Delay1/1, Sum3/2
  Compare To Constant/1 -> Switch/2
  Abs/1 -> Compare To Constant/1
  Gin3/1 -> Switch/3  "w(k)"
  Gin4/1 -> Switch/1  "w(k-1)"
  Sum1/1 -> Gin3/1, Abs/1
  Sum/1 -> Gin4/1
  Unit Delay2/1 -> Sum/1  "eCountR(k-2)"
  Unit Delay/1 -> Sum1/1, Sum/2, Unit Delay2/1  "eCountR(k-1)"
  eCountR/1 -> Sum1/2, Unit Delay/1

== system track_vehicle_EKF1/GNC/Guidance2/Subsystem1/Triggered Subsystem2 ==
  Trigger : TriggerPort  VariantControl=(inherit)
  Constant : Constant  OutDataTypeStr=uint32  SampleTime=-1
  Out1 : Outport  OutDataTypeStr=uint32  InitialOutput=0
  wires:
  Constant/1 -> Out1/1

== system track_vehicle_EKF1/GNC/Guidance2/Unwrap Angle/Triggered Subsystem ==
  Trigger : TriggerPort  VariantControl=(inherit)
  Sum3 : Sum  OutDataTypeStr=int32
  Unit Delay : UnitDelay  SampleTime=-1
  countIncrement : Constant  OutDataTypeStr=int32  SampleTime=-1
  Out1 : Outport  OutDataTypeStr=int32  InitialOutput=0
  wires:
  countIncrement/1 -> Sum3/2
  Unit Delay/1 -> Sum3/1
  Sum3/1 -> Out1/1, Unit Delay/1

== system track_vehicle_EKF1/GNC/Guidance2/Unwrap Angle/Triggered Subsystem1 ==
  Trigger : TriggerPort  VariantControl=(inherit)
  Sum3 : Sum  Inputs=+-  OutDataTypeStr=int32
  Unit Delay : UnitDelay  SampleTime=-1
  countIncrement : Constant  OutDataTypeStr=int32  SampleTime=-1
  Out1 : Outport  OutDataTypeStr=int32  InitialOutput=0
  wires:
  Sum3/1 -> Out1/1, Unit Delay/1
  Unit Delay/1 -> Sum3/1
  countIncrement/1 -> Sum3/2

== matlab function track_vehicle_EKF1/GNC/Navigation (DeadReckoning)/Kalman Filter ==
  data: xGPS input; yGPS input; thetaCompass input; VGPS input; omegaGyro input; wL input; wR input; st output; Tsample parameter; rNominalDR parameter; bDR parameter; covv output
function [st,covv] =  ExtKalman(xGPS,yGPS,thetaCompass,VGPS,omegaGyro,wL,wR,Tsample,rNominalDR,bDR)
%#codegen


meas=[xGPS;yGPS;thetaCompass;VGPS;omegaGyro];
persistent P xhat 
if isempty(P)
   % First time through the code so do some initialization
   xhat = zeros(5,1);
   P = zeros(5,5);
 end 
   Q = diag([0.003 0.005 0.0145 0.01165161 0]);     % odometry cov 
   %Q = diag([1.3329 0.7887 0.0145 0.01165161 1.34E-08]);
   R = diag([1.3329 0.7887 0.0145 0.01165161 1.34E-08]);
   %R = 150*diag([0.6009 1.0176 0.3438 0.006661 3.56e-08]);
  % R = 150*diag([1 1 1 1 1]);
   
% Calculate the Jacobians for the state and measurement equations
F = [1 0  -Tsample*xhat(4)*sin(xhat(3)) Tsample*cos(xhat(3)) 0 ;
     0 1   Tsample*xhat(4)*cos(xhat(3)) Tsample*sin(xhat(3)) 0 ;
     0 0            1                 0           Tsample ;
     0 0            0                 0            0 ;
     0 0            0                 0            0 ];
H =eye(5);
% Propogate  the state and covariance matrices
xhat = [...
    xhat(1) + Tsample*xhat(4)*cos(xhat(3));
    xhat(2) + Tsample*xhat(4)*sin(xhat(3));
    xhat(3)  + Tsample * xhat(5);
    rNominalDR*(wL+wR)/2;
    rNominalDR*(wL-wR)/bDR];


P = F*P*F' + Q;
% Calculate the Kalman gain
K = P*H'/(H*P*H' + R);
% Calculate the measurement residual
yhat = H*xhat;
resid = meas - yhat;
% Update the state and covariance estimates
xhat = xhat + K*resid;
P = (eye(size(K,1))-K*H)*P;
% Post the results
st = xhat;
covv = P;

== matlab function track_vehicle_EKF1/GNC/Guidance2/MATLAB Function ==
  data: Range input; angleAvoid output
function angleAvoid = fcn(Range)

if Range <=1.5 && Range >= 0.21
    angleAvoid=-13*pi/36;
else
    angleAvoid=0;

end
